simulink model "W06_Rlocus_Verify"  (R2024b)
settings: Solver=ode45  StartTime=0.0  StopTime=t_end  MaxStep=0.005  RelTol=1e-3
PreLoadFcn:
  | % W06_Rlocus_Verify 기본 파라미터 (모델을 열 때 자동 실행)
  | % u_lim 이 크므로 기본 상태는 포화 없음 = 선형 이론과 같은 결과
  | defs = { 'K',30 ; 'r_amp',1 ; 'u_lim',1e6 ; 't_end',6 ;
  |          'numG',0.01 ; 'denG',[0.005 0.06 0.1001 0] };
  | for ii = 1:size(defs,1)
  |     if ~evalin('base', sprintf('exist(''%s'',''var'')', defs{ii,1}))
  |         assignin('base', defs{ii,1}, defs{ii,2});
  |     end
  | end
  | clear defs ii
values from neighbouring files (symbols this model uses):
  K = 20    [W06_03_run_simulink.m]
  r_amp = 1    [W06_03_run_simulink.m]
  u_lim = u_limits(i)    [W06_03_run_simulink.m]
undefined symbols (not defined in the file or in its folder): denG, numG
settings Model: Creator=admin  LastModifiedBy=admin

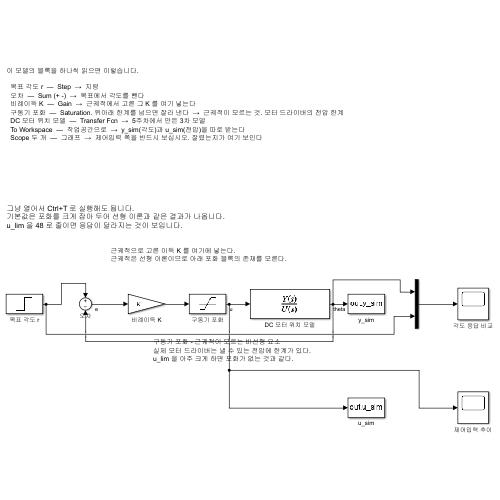
[thumbnail: Simulink's stored preview of the top-level diagram]
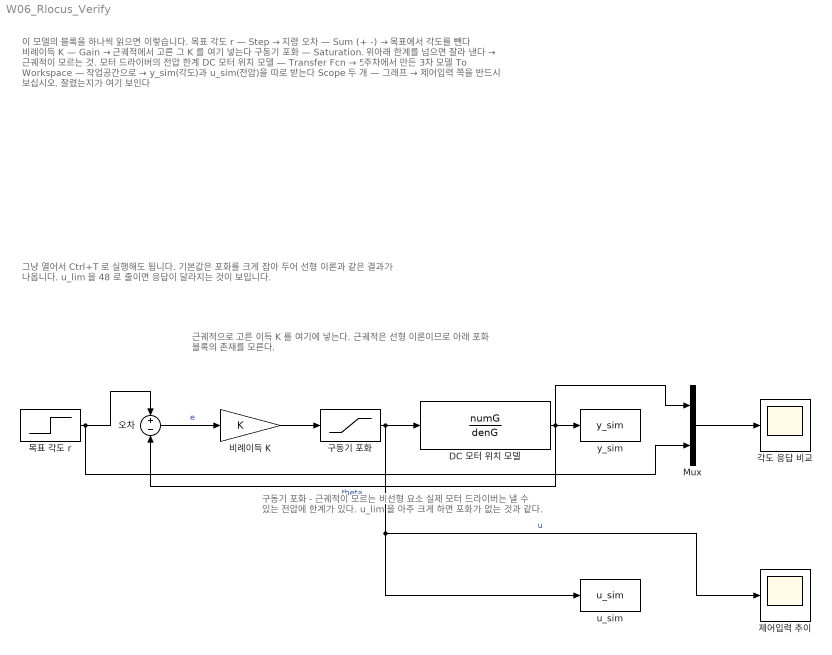
== system W06_Rlocus_Verify ==
  note: 근궤적으로 고른 이득 K 를 여기에 넣는다.
      | 근궤적은 선형 이론이므로 아래 포화 블록의 존재를 모른다.
  note: 구동기 포화 - 근궤적이 모르는 비선형 요소
      | 실제 모터 드라이버는 낼 수 있는 전압에 한계가 있다.
      | u_lim 을 아주 크게 하면 포화가 없는 것과 같다.
  note: 그냥 열어서 Ctrl+T 로 실행해도 됩니다.
      | 기본값은 포화를 크게 잡아 두어 선형 이론과 같은 결과가 나옵니다.
      | u_lim 을 48 로 줄이면 응답이 달라지는 것이 보입니다.
  note: 이 모델의 블록을 하나씩 읽으면 이렇습니다.
      |
      |   목표 각도 r  —  Step  →  지령
      |   오차  —  Sum (+ -)  →  목표에서 각도를 뺀다
      |   비례이득 K  —  Gain  →  근궤적에서 고른 그 K 를 여기 넣는다
      |   구동기 포화  —  Saturation. 위아래 한계를 넘으면 잘라 낸다  →  근궤적이 모르는 것. 모터 드라이버의 전압 한계
      |   DC 모터 위치 모델  —  Transfer Fcn  →  5주차에서 만든 3차 모델
      |   To Workspace  —  작업공간으로  →  y_sim(각도)과 u_sim(전압)을 따로 받는다
      |   Scope 두 개  —  그래프  →  제어입력 쪽을 반드시 보십시오. 잘렸는지가 여기 보인다
  DC 모터 위치 모델 : TransferFcn  Numerator=numG  Denominator=denG
  Mux : Mux  Inputs=2
  u_sim : ToWorkspace  VariableName=u_sim  SaveFormat=Timeseries  SampleTime=-1
  y_sim : ToWorkspace  VariableName=y_sim  SaveFormat=Timeseries  SampleTime=-1
  각도 응답 비교 : Scope
  구동기 포화 : Saturate  UpperLimit=u_lim  LowerLimit=-u_lim
  목표 각도 r : Step  Time=0  After=r_amp  SampleTime=0
  비례이득 K : Gain  Gain=K
  오차 : Sum  Inputs=+-
  제어입력 추이 : Scope
  wires:
  목표 각도 r/1 -> 오차/1, Mux/2
  오차/1 -> 비례이득 K/1  "e"
  비례이득 K/1 -> 구동기 포화/1
  구동기 포화/1 -> u_sim/1, 제어입력 추이/1, DC 모터 위치 모델/1  "u"
  DC 모터 위치 모델/1 -> y_sim/1, 오차/2, Mux/1  "theta"
  Mux/1 -> 각도 응답 비교/1
